simulink model "test_EN12977_StorageType1_Strat"  (Simulink 8.2)
settings: Solver=ode45  StartTime=time(1)  StopTime=time(end)  MaxStep=time(2)-time(1)  RelTol=1e-3
values from neighbouring files (symbols this model uses):
  Tstg = [0 10 20 30 40 50 60 70 80 90 100 110 ... (32417 elements, 2947x11)]    [data_EN12977_sequence_C.mat]    (also in data_EN12977_sequence_CD.mat = [0 10 20 30 40 50 60 70 80 90 100 110 ... (221958 elements, ; data_EN12977_sequence_DD.mat = [0 10 20 30 40 50 60 70 80 90 100 110 ... (25608 elements, 2; data_EN12977_sequence_NA.mat = [0 10 20 30 40 50 60 70 80 90 100 110 ... (20834 elements, 1; data_EN12977_sequence_NB.mat = [0 10 20 30 40 50 60 70 80 90 100 110 ... (115929 elements, )
libraries: carnot x19
settings Model: Creator=drhf  LastModifiedBy=drhf
settings DataIOCC: SaveOutput=off  SaveTime=off

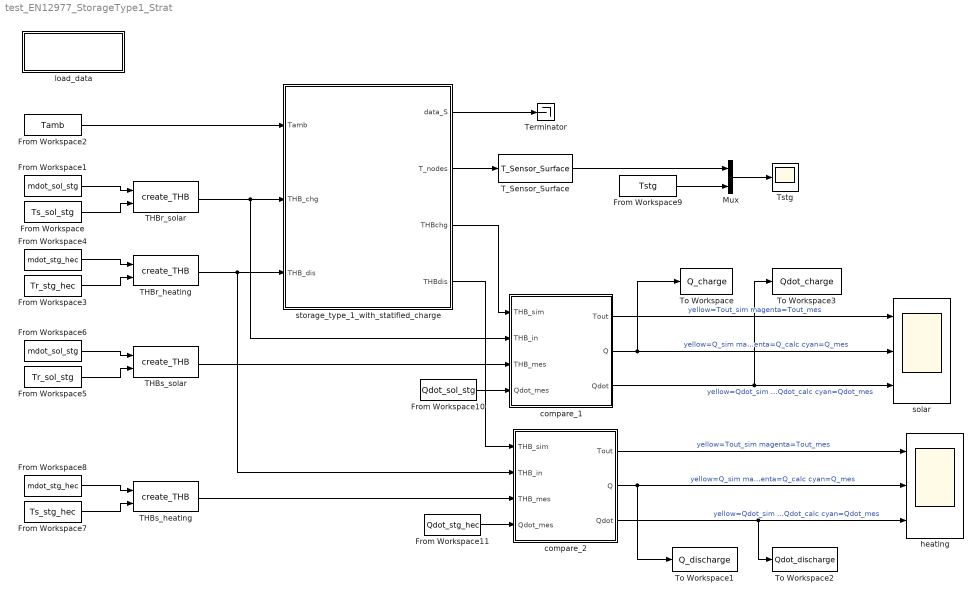
== system test_EN12977_StorageType1_Strat ==
  From Workspace : FromWorkspace  VariableName=Ts_sol_stg  SampleTime=0
  From Workspace1 : FromWorkspace  VariableName=mdot_sol_stg  SampleTime=0
  From Workspace10 : FromWorkspace  VariableName=Qdot_sol_stg  SampleTime=0
  From Workspace11 : FromWorkspace  VariableName=Qdot_stg_hec  SampleTime=0
  From Workspace2 : FromWorkspace  VariableName=Tamb  SampleTime=0
  From Workspace3 : FromWorkspace  VariableName=Tr_stg_hec  SampleTime=0
  From Workspace4 : FromWorkspace  VariableName=mdot_stg_hec  SampleTime=0
  From Workspace5 : FromWorkspace  VariableName=Tr_sol_stg  SampleTime=0
  From Workspace6 : FromWorkspace  VariableName=mdot_sol_stg  SampleTime=0
  From Workspace7 : FromWorkspace  VariableName=Ts_stg_hec  SampleTime=0
  From Workspace8 : FromWorkspace  VariableName=mdot_stg_hec  SampleTime=0
  From Workspace9 : FromWorkspace  VariableName=Tstg  SampleTime=0
  Mux : Mux  Inputs=2
  THBr_heating : carnot/Source/Simple/create_THB  p=1e5  fluid=Water  mix=0  dia=0.02  mID=No Pressure Drop
  THBr_solar : carnot/Source/Simple/create_THB  p=1e5  fluid=Water  mix=0  dia=0.02  mID=No Pressure Drop
  THBs_heating : carnot/Source/Simple/create_THB  p=1e5  fluid=Water  mix=0  dia=0.02  mID=No Pressure Drop
  THBs_solar : carnot/Source/Simple/create_THB  p=1e5  fluid=Water  mix=0  dia=0.02  mID=No Pressure Drop
  T_Sensor_Surface : carnot/Control/T_Sensor_Surface  pos=[0.8830 0.7980 0.7130 0.6280 0.5430 0.4570 0.3720 0.2870 0.2020 0.1170]  tdel=1  t0=Tstg(1, 2:11)
  Terminator : Terminator
  To Workspace : ToWorkspace  VariableName=Q_charge  SampleTime=-1
      settings: MaxDataPoints=1
  To Workspace1 : ToWorkspace  VariableName=Q_discharge  SampleTime=-1
      settings: MaxDataPoints=1
  To Workspace2 : ToWorkspace  VariableName=Qdot_discharge  SampleTime=180
  To Workspace3 : ToWorkspace  VariableName=Qdot_charge  SampleTime=180
  Tstg : Scope
      settings: YMin=15  YMax=60  SaveName=ScopeData5
  compare_1 : Subsystem
  compare_2 : Subsystem
  heating : Scope  NumInputPorts=3
      settings: YMin=20~-4e+007~-7500  YMax=60~4e+007~7500  SaveName=ScopeData4
  load_data : Subsystem
      settings: OpenFcn=|
      | [filename, pathname, filterindex] = ...
      |    uigetfile( {  'data*.mat', ...
      |    'validation files (data*.mat)'; ...
      |    '*.mat','MAT-files (*.mat)'; ...
      |    '*.*',  'All Files (*.*)'},  'Pick a data file');
      | 
      | if (filterindex > 0)
      |    load(filename)
      | end
      mask Display: disp('double click \nto load data')
  solar : Scope  NumInputPorts=3
      settings: YMin=17.5~-1.9e+007~-5500  YMax=60~1e+006~4500  SaveName=ScopeData2
  storage_type_1_with_statified_charge : Subsystem  mask(Multiport Storage){uloss=1.4, ubot=1.4, utop=1.4, cond=1.2, tini=interp1(1:10, Tstg(1, 2:end), 10:-9/99:1), volume=0.225, dia=0.53, pos=standing cylinder, nconnect=2, nodes=100, mpoints=100}
      mask prompts: uloss "Heat loss coefficient cylinder wall in W/(m²K)"; ubot "Heat loss coefficient bottom in W/(m²K)"; utop "Heat loss coefficient top cover in W/(m²K)"; cond "Effective vertical conductivity in W/(m*K)"; tini "Initial temperature (vector or scalar) in °C"; volume "Volume in m³"; dia "Diameter in m"; pos "Position"; nconnect "Number of connections"; nodes "Number of nodes"; mpoints "Number of measurement points"
      mask help:
      | The volmue of the cylindrical storage is divided in a number "nodes" of horizontal slices (1xN-node model). For each node the energy balance equation is solved.
      | Look under mask to set the ports types and properties.
      mask init:
      | standing = pos-1;
      | 
      | if standing
      |     dh = volume/(0.25*dia^2*pi*nodes);
      | else
      |     dh = dia/nodes;
      | end
      | 
      | % height = 0.5*dh : dh : dh*nodes;
      | height = dh*nodes;
      | 
      | mpoints = max(mpoints,1);
      | mpts = round(nodes/mpoints/2:nodes/mpoints:nodes);
      mask Help: eval('man(''storage_multiport'')')
      mask TypeOptions pos: lying cylinder | standing cylinder
      mask Display: plot(10,10,90,100,[40,40,45,55,60,60,55,45,40],[84,36,30,30,36,84,90,90,84],[40,35],[77,77],[64,60],[77,77],[40,35],[42,42],[64,60],[42,42])
  wires:
  storage_type_1_with_statified_charge/1(data_S) -> Terminator/1
  storage_type_1_with_statified_charge/2(T_nodes) -> T_Sensor_Surface/1
  From Workspace2/1 -> storage_type_1_with_statified_charge/1(Tamb)
  THBr_solar/1 -> compare_1/2(THB_in), storage_type_1_with_statified_charge/2(THB_chg)
  THBr_heating/1 -> storage_type_1_with_statified_charge/3(THB_dis), compare_2/2(THB_in)
  compare_1/1(Tout) -> solar/1  "yellow=Tout_sim magenta=Tout_mes"
  compare_1/2(Q) -> solar/2, To Workspace/1  "yellow=Q_sim magenta=Q_calc cyan=Q_mes"
  storage_type_1_with_statified_charge/3(THBchg) -> compare_1/1(THB_sim)
  THBs_solar/1 -> compare_1/3(THB_mes)
  compare_2/1(Tout) -> heating/1  "yellow=Tout_sim magenta=Tout_mes"
  compare_2/2(Q) -> heating/2, To Workspace1/1  "yellow=Q_sim magenta=Q_calc cyan=Q_mes"
  THBs_heating/1 -> compare_2/3(THB_mes)
  storage_type_1_with_statified_charge/4(THBdis) -> compare_2/1(THB_sim)
  Mux/1 -> Tstg/1
  T_Sensor_Surface/1 -> Mux/1
  From Workspace9/1 -> Mux/2
  compare_1/3(Qdot) -> solar/3, To Workspace3/1  "yellow=Qdot_sim magenta=Qdot_calc cyan=Qdot_mes"
  From Workspace10/1 -> compare_1/4(Qdot_mes)
  From Workspace11/1 -> compare_2/4(Qdot_mes)
  compare_2/3(Qdot) -> heating/3, To Workspace2/1  "yellow=Qdot_sim magenta=Qdot_calc cyan=Qdot_mes"
  From Workspace1/1 -> THBr_solar/1
  From Workspace/1 -> THBr_solar/2
  From Workspace4/1 -> THBr_heating/1
  From Workspace3/1 -> THBr_heating/2
  From Workspace6/1 -> THBs_solar/1
  From Workspace5/1 -> THBs_solar/2
  From Workspace8/1 -> THBs_heating/1
  From Workspace7/1 -> THBs_heating/2

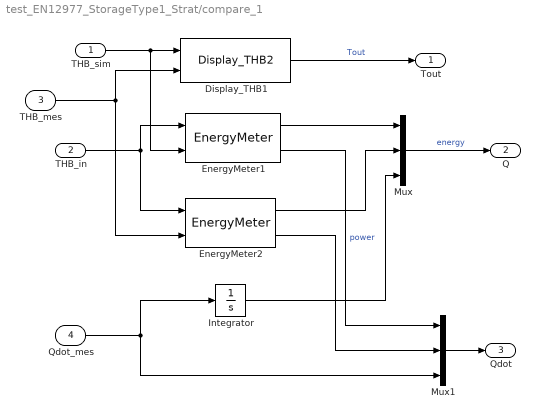
== system test_EN12977_StorageType1_Strat/compare_1 ==
  THB_sim : Inport
  THB_in : Inport  Port=2
  THB_mes : Inport  Port=3
  Qdot_mes : Inport  Port=4
  Display_THB1 : carnot/Outputs/Display_THB2  t=on  m=off  p=off  id=off  mix=off  d=off
  EnergyMeter1 : carnot/Control/EnergyMeter
  EnergyMeter2 : carnot/Control/EnergyMeter
  Integrator : Integrator  UpperSaturationLimit=1  LowerSaturationLimit=0
  Mux : Mux  Inputs=3
  Mux1 : Mux  Inputs=3
  Tout : Outport
  Q : Outport  Port=2
  Qdot : Outport  Port=3
  wires:
  THB_sim/1 -> EnergyMeter1/2, Display_THB1/1
  THB_mes/1 -> EnergyMeter2/2, Display_THB1/2
  EnergyMeter1/1 -> Mux/1
  Display_THB1/1 -> Tout/1  "Tout"
  Mux/1 -> Q/1  "energy"
  Qdot_mes/1 -> Integrator/1, Mux1/3
  EnergyMeter1/2 -> Mux1/1  "power"
  Mux1/1 -> Qdot/1
  THB_in/1 -> EnergyMeter2/1, EnergyMeter1/1
  EnergyMeter2/1 -> Mux/2
  EnergyMeter2/2 -> Mux1/2
  Integrator/1 -> Mux/3

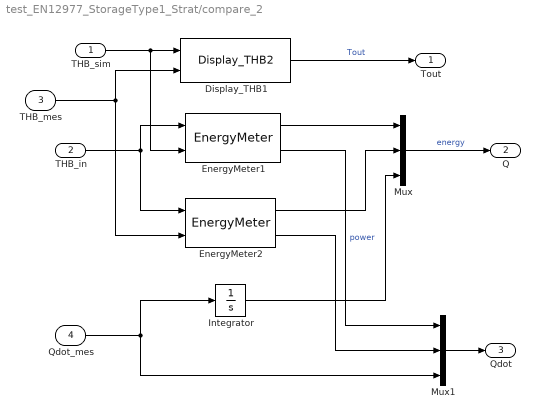
== system test_EN12977_StorageType1_Strat/compare_2 ==
  THB_sim : Inport
  THB_in : Inport  Port=2
  THB_mes : Inport  Port=3
  Qdot_mes : Inport  Port=4
  Display_THB1 : carnot/Outputs/Display_THB2  t=on  m=off  p=off  id=off  mix=off  d=off
  EnergyMeter1 : carnot/Control/EnergyMeter
  EnergyMeter2 : carnot/Control/EnergyMeter
  Integrator : Integrator  UpperSaturationLimit=1  LowerSaturationLimit=0
  Mux : Mux  Inputs=3
  Mux1 : Mux  Inputs=3
  Tout : Outport
  Q : Outport  Port=2
  Qdot : Outport  Port=3
  wires:
  Integrator/1 -> Mux/3
  EnergyMeter2/2 -> Mux1/2
  EnergyMeter2/1 -> Mux/2
  THB_in/1 -> EnergyMeter1/1, EnergyMeter2/1
  Mux1/1 -> Qdot/1
  EnergyMeter1/2 -> Mux1/1  "power"
  Qdot_mes/1 -> Mux1/3, Integrator/1
  Mux/1 -> Q/1  "energy"
  Display_THB1/1 -> Tout/1  "Tout"
  EnergyMeter1/1 -> Mux/1
  THB_mes/1 -> Display_THB1/2, EnergyMeter2/2
  THB_sim/1 -> Display_THB1/1, EnergyMeter1/2

== system test_EN12977_StorageType1_Strat/load_data ==

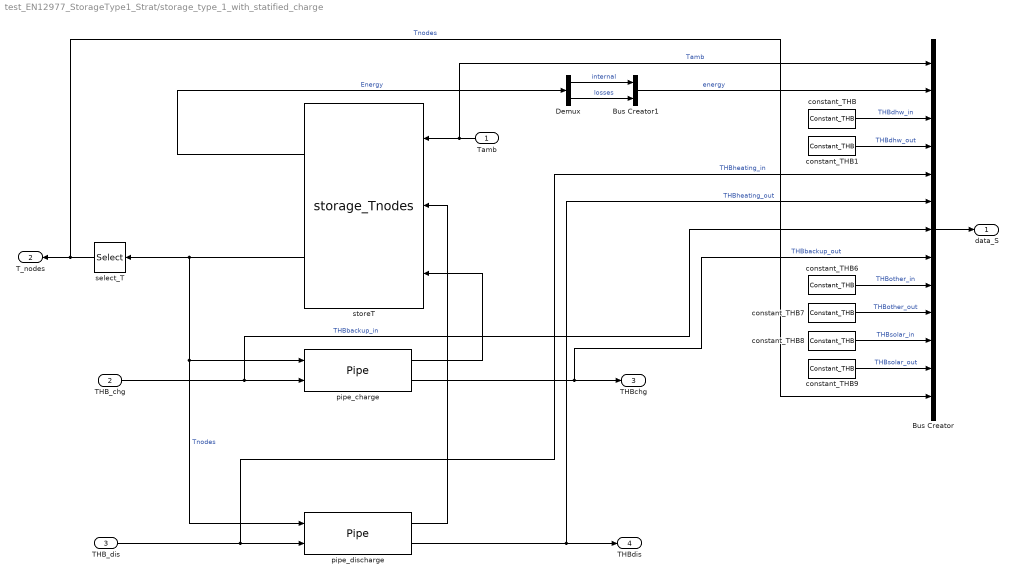
== system test_EN12977_StorageType1_Strat/storage_type_1_with_statified_charge ==
  Tamb : Inport
  THB_chg : Inport  Port=2
  THB_dis : Inport  Port=3
  Bus Creator : BusCreator  Inputs=13
  Bus Creator1 : BusCreator  Inputs=2
  Demux : Demux  Outputs=2
  constant_THB{,1,6..9} (6 alike) : carnot/Source/Simple/Constant_THB  t=20  mdot=0  p=1e5  mID=No Pressure Drop  fluid=Water  mix=0  dia=0.02  hgt=0
  pipe_charge : carnot/Storage/Thermal/Storage_Ports/Pipe  h_in=0.62  h_out=0  dplin=0  dpqua=0  nodes=nodes  hgt=height  dia=dia
  pipe_discharge : carnot/Storage/Thermal/Storage_Ports/Pipe  h_in=0.1  h_out=1  dplin=0  dpqua=0  nodes=nodes  hgt=height  dia=dia
  select_T : Selector  InputPortWidth=nodes  IndexOptions=Index vector (dialog)  Indices=mpts  OutputSizes=1
  storeT : S-Function  FunctionName=storage_Tnodes  Parameters=dia, volume, standing, uloss , ubot, utop, cond, tini, nodes, nconnect  EnableBusSupport=off
  data_S : Outport
  T_nodes : Outport  Port=2
  THBchg : Outport  Port=3
  THBdis : Outport  Port=4
  wires:
  Tamb/1 -> storeT/1, Bus Creator/1  "Tamb"
  THB_dis/1 -> Bus Creator/5, pipe_discharge/2  "THBheating_in"
  pipe_discharge/2 -> THBdis/1, Bus Creator/6  "THBheating_out"
  pipe_discharge/1 -> storeT/2
  select_T/1 -> T_nodes/1, Bus Creator/13  "Tnodes"
  storeT/1 -> Demux/1  "Energy"
  storeT/2 -> select_T/1, pipe_charge/1, pipe_discharge/1  "Tnodes"
  constant_THB1/1 -> Bus Creator/4  "THBdhw_out"
  constant_THB/1 -> Bus Creator/3  "THBdhw_in"
  Bus Creator/1 -> data_S/1
  constant_THB9/1 -> Bus Creator/12  "THBsolar_out"
  constant_THB8/1 -> Bus Creator/11  "THBsolar_in"
  constant_THB7/1 -> Bus Creator/10  "THBother_out"
  constant_THB6/1 -> Bus Creator/9  "THBother_in"
  THB_chg/1 -> Bus Creator/7, pipe_charge/2  "THBbackup_in"
  pipe_charge/2 -> THBchg/1, Bus Creator/8  "THBbackup_out"
  pipe_charge/1 -> storeT/3
  Demux/1 -> Bus Creator1/1  "internal"
  Demux/2 -> Bus Creator1/2  "losses"
  Bus Creator1/1 -> Bus Creator/2  "energy"
